simulink model "gxx"  (R2016b)
settings: Solver=VariableStepAuto  StartTime=0.0  StopTime=76  EnableMultiTasking=on
InitFcn:
  | run('motor_param.m')
values from neighbouring files (symbols this model uses):
  battery_Voltage = 390.4254    [motor_param.m]
  Damp = 4.1785e-04    (= 0.00041785)    [motor_param.m]
  Damperr = 0.001    [motor_param.m]
  Inrt = 2.500893701670255e-04    (= 0.000250089370167)    [motor_param.m]
  Pole_pairs = 3    [motor_param.m]
  resistance = 0.11607    [motor_param.m]
  stator_phase_resistance = 0.049039279360294    (= 0.0490392793603)    [motor_param.m]
  temp_amb = 27+273    (= 300)    [motor_param.m]
  Ts = 1e-4    (= 0.0001)    [motor_param.m]
undefined symbols (not defined in the file or in its folder): mot
libraries: fl_lib x17, nesl_utility x8, powerlib x8, simulink x4, electricdrivelib x2, spsDrivesPrivateModels x1
settings Model: Creator=thepu  LastModifiedBy=gd7198
settings OptimizationCC: LifeSpan=inf
settings DebuggingCC: SFUnexpectedBacktrackingDiag=warning  SFNoUnconditionalDefaultTransitionDiag=warning  SFExecutionAtInitializationDiag=none
settings GRTTargetCC: TargetLangStandard=C89/C90 (ANSI)  GeneratePreprocessorConditionals=Disable all
settings ConfigComp: CovMetricSettings=dw  CovHtmlReporting=on  CovSaveCumulativeToWorkspaceVar=on  CovSaveSingleToWorkspaceVar=on  CovExternalEMLEnable=off

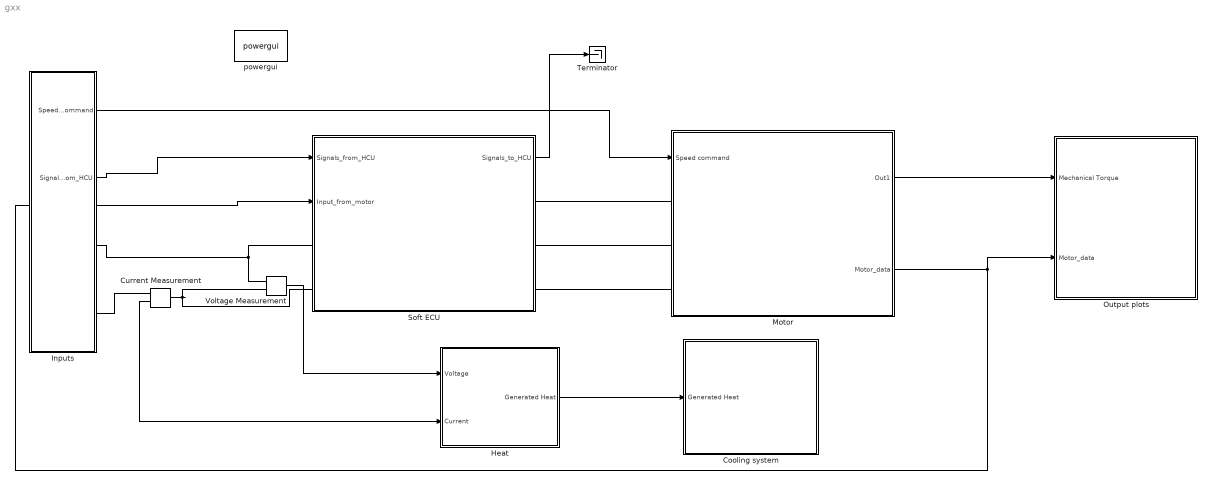
== system gxx ==
  Cooling system : Subsystem
  Current Measurement : powerlib/Measurements/Current Measurement  PhasorSimulation=off  OutputType=Complex  PSBequivalent=0
  Heat : Subsystem
  Inputs : Subsystem
  "Motor " : Subsystem
  Output plots : Subsystem
  Soft ECU : Subsystem
  Terminator : Terminator
  Voltage Measurement : powerlib/Measurements/Voltage Measurement  PhasorSimulation=off  OutputType=Complex  PSBequivalent=0
  powergui : powerlib/powergui  Priority=1  SimulationMode=Discrete  SolverType=Backward Euler  SampleTime=Ts  frequency=60  SPID=off  DisableSnubberDevices=off  DisableRonSwitches=off  DisableVfSwitches=off  SwTol=0  DisplayEquations=off  Interpol=on  ExternalGateDelay=off  methode=off  Ts=10  FunctionMessages=off  echomessages=off  HookPort=off  EnableUseOfTLC=off  x0status=blocks  frequencyindice=0  Pbase=100e6  ErrMax=1e-4  Iterations=50  UnitsV=kV  UnitsW=MW  buscounter=0  RestoreLinks=warning  ResistiveCurrentMeasurement=off  Frange=[0:2:500]  Ylog=off  Xlog=on  ShowGrid=off  save=off  variable=ZData  structure=0  ZoomFFT=off  StartTime=0.0  cycles=1  DisplayStyle=1  fundamental=60  FreqAxis=off  MaxFrequency=1000  frequencyindicesteady=1  RmsSteady=1  display=off
  wires:
  "Motor "/2(Motor_data) -> Soft ECU/2(Input_from_motor), Output plots/2(Motor_data)
  Heat/1(Generated Heat) -> Cooling system/1(Generated Heat)
  Inputs/1(Speed_command) -> "Motor "/1(Speed command)
  "Motor "/1(Out1) -> Output plots/1(Mechanical Torque)
  Inputs/2(Signals_From_HCU) -> Soft ECU/1(Signals_from_HCU)
  Soft ECU/1(Signals_to_HCU) -> Terminator/1
  Voltage Measurement/1 -> Heat/1(Voltage)
  Current Measurement/1 -> Heat/2(Current)
  connections:
  Inputs/RConn1 -- Voltage Measurement/LConn1 -- Soft ECU/LConn1
  "Motor "/LConn1 -- Soft ECU/RConn1
  Soft ECU/RConn2 -- "Motor "/LConn2
  Soft ECU/RConn3 -- "Motor "/LConn3
  Current Measurement/LConn1 -- Voltage Measurement/LConn2 -- Soft ECU/LConn2
  Current Measurement/RConn1 -- Inputs/RConn2

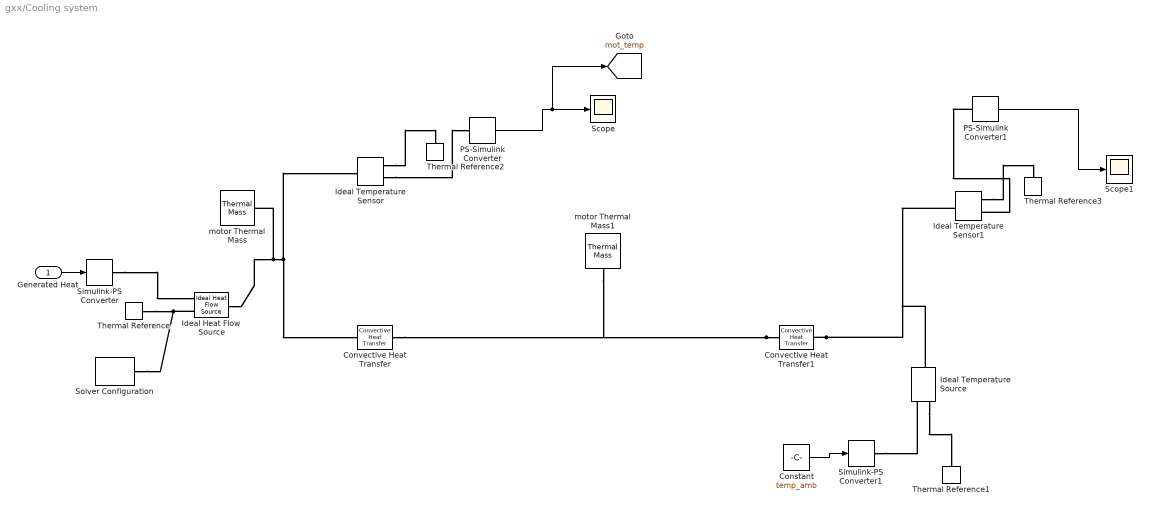
== system gxx/Cooling system ==
  Generated Heat : Inport
  Constant : Constant  Value=temp_amb
  Convective Heat Transfer : fl_lib/Thermal/Thermal Elements/Convective Heat Transfer  area=htArea m^2  heat_tr_coeff=hcm W/(m^2 * K)  Q_specify=off  Q_priority=None  Q=0 J/s  T_specify=off  T_priority=None  T=0 K
  Convective Heat Transfer1 : fl_lib/Thermal/Thermal Elements/Convective Heat Transfer  area=radiator_area m^2  heat_tr_coeff=hac W/(m^2 * K)  Q_specify=off  Q_priority=None  Q=0 J/s  T_specify=off  T_priority=None  T=0 K
  Ideal Heat Flow Source : fl_lib/Thermal/Thermal Sources/Ideal Heat Flow Source
  Ideal Temperature Sensor : fl_lib/Thermal/Thermal Sensors/Ideal Temperature Sensor
  Ideal Temperature Sensor1 : fl_lib/Thermal/Thermal Sensors/Ideal Temperature Sensor
  Ideal Temperature Source : fl_lib/Thermal/Thermal Sources/Ideal Temperature Source
  PS-Simulink Converter : nesl_utility/PS-Simulink Converter  PhysicalDomain=network_engine_domain  SubClassName=ps_output  LeftPortType=input  RightPortType=output  PseudoPeriodic=off  Frequencies=[]  Unit=K  AffineConversion=off
  PS-Simulink Converter1 : nesl_utility/PS-Simulink Converter  PhysicalDomain=network_engine_domain  SubClassName=ps_output  LeftPortType=input  RightPortType=output  PseudoPeriodic=off  Frequencies=[]  Unit=K  AffineConversion=off
  Scope : Scope
  Scope1 : Scope
  Simulink-PS Converter : nesl_utility/Simulink-PS Converter  PhysicalDomain=network_engine_domain  SubClassName=ps_input  LeftPortType=input  RightPortType=output  PseudoPeriodic=off  Frequencies=[]  NoiseDistribution=none  NoiseParameters=[]  Unit=1  AffineConversion=off  InputFiltering=off  SimscapeFilterOrder=1  InputFilterTimeConstant=0.001  UdotUserProvided=1
  Simulink-PS Converter1 : nesl_utility/Simulink-PS Converter  PhysicalDomain=network_engine_domain  SubClassName=ps_input  LeftPortType=input  RightPortType=output  PseudoPeriodic=off  Frequencies=[]  NoiseDistribution=none  NoiseParameters=[]  Unit=K  AffineConversion=off  InputFiltering=off  SimscapeFilterOrder=1  InputFilterTimeConstant=0.001  UdotUserProvided=1
  Solver Configuration : nesl_utility/Solver Configuration  PhysicalDomain=network_engine_domain  SubClassName=solver  LeftPortType=input  RightPortType=generic  Accelerate=off  Tones=[]  Harmonics=[]  SimulateNoise=off  Profile=off  UseLocalSampling=off  EnableSwitchedLinearOptims=on  FrequencyDomain=off  UseCCode=off  RelTol=0.001  AbsTol=1e-06  MinStep=1e-09  ToWorkspace=off  RevertToSquareIcSolve=off  NumHomotopyIterations=100  PhasorMode=off  PhasorModeNumHarmonics=1  OverrideAbsTol=off  DoDC=off  ResidualTolerance=1e-9  UseLocalSolver=off  LocalSolverChoice=NE_BACKWARD_EULER_ADVANCER  LocalSolverSampleTime=0.1  DoFixedCost=off  MaxNonlinIter=3  MaxModeIter=2  LinearAlgebra=Sparse  DelaysMemoryBudget=1024  AutomaticFiltering=on  FilteringTimeConstant=0.001
  Thermal Reference{,1..3} (4 alike) : fl_lib/Thermal/Thermal Elements/Thermal Reference
  motor Thermal Mass : fl_lib/Thermal/Thermal Elements/Thermal Mass  mass=motor_mass kg  sp_heat=motor_cp J/kg/K  T_specify=on  T_priority=High  T=temp_amb K  Q_specify=off  Q_priority=High  Q=0 J/s
  motor Thermal Mass1 : fl_lib/Thermal/Thermal Elements/Thermal Mass  mass=coolant_mass kg  sp_heat=coolant_cp J/kg/K  T_specify=on  T_priority=High  T=temp_amb degC  Q_specify=off  Q_priority=High  Q=0 J/s
  tag scope: mot_temp=global
  wires:
  Generated Heat/1 -> Simulink-PS Converter/1
  Constant/1 -> Simulink-PS Converter1/1
  PS-Simulink Converter/1 -> [mot_temp], Scope/1
  PS-Simulink Converter1/1 -> Scope1/1
  connections:
  Thermal Reference/LConn1 -- Solver Configuration/RConn1 -- Ideal Heat Flow Source/RConn2
  Ideal Heat Flow Source/LConn1 -- motor Thermal Mass/LConn1 -- Ideal Temperature Sensor/LConn1 -- Convective Heat Transfer/LConn1
  Simulink-PS Converter/RConn1 -- Ideal Heat Flow Source/RConn1
  Convective Heat Transfer1/LConn1 -- Convective Heat Transfer/RConn1 -- motor Thermal Mass1/LConn1
  Convective Heat Transfer1/RConn1 -- Ideal Temperature Source/LConn1 -- Ideal Temperature Sensor1/LConn1
  Simulink-PS Converter1/RConn1 -- Ideal Temperature Source/RConn1
  Ideal Temperature Source/RConn2 -- Thermal Reference1/LConn1
  Ideal Temperature Sensor/RConn1 -- Thermal Reference2/LConn1
  Ideal Temperature Sensor/RConn2 -- PS-Simulink Converter/LConn1
  Ideal Temperature Sensor1/RConn1 -- Thermal Reference3/LConn1
  PS-Simulink Converter1/LConn1 -- Ideal Temperature Sensor1/RConn2

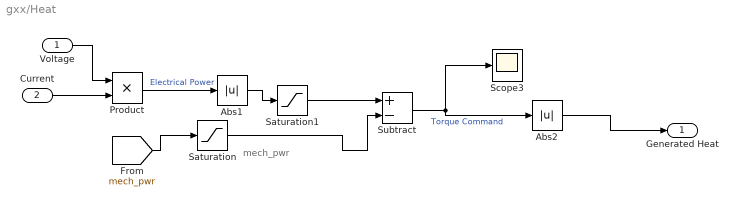
== system gxx/Heat ==
  note: mech_pwr
  Voltage : Inport
  Current : Inport  Port=2
  Abs1 : Abs
  Abs2 : Abs
  Product : Product
  Saturation : Saturate  UpperLimit=100000  LowerLimit=-100000
  Saturation1 : Saturate  UpperLimit=1000000  LowerLimit=-1000000
  Scope3 : Scope
  Subtract : Sum  Inputs=+-
  Generated Heat : Outport
  wires:
  Voltage/1 -> Product/1
  [mech_pwr] -> Saturation/1
  Abs1/1 -> Saturation1/1
  Product/1 -> Abs1/1  "Electrical Power"
  Saturation/1 -> Subtract/2
  Subtract/1 -> Scope3/1, Abs2/1  "Torque Command"
  Abs2/1 -> Generated Heat/1
  Saturation1/1 -> Subtract/1
  Current/1 -> Product/2

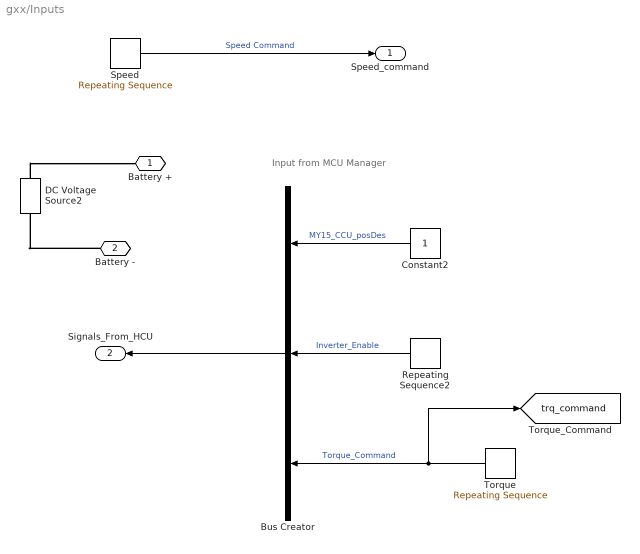
== system gxx/Inputs ==
  note: Input from MCU Manager
  Bus Creator : BusCreator  Inputs=3
  Constant2 : Constant
  DC Voltage Source2 : powerlib/Electrical Sources/DC Voltage Source  Amplitude=battery_Voltage  Measurements=Voltage
  Repeating Sequence2 : simulink/Sources/Repeating Sequence  rep_seq_t=time_test  rep_seq_y=inverterEnable
  Speed : simulink/Sources/Repeating Sequence  rep_seq_t=time_test  rep_seq_y=spd_command
  Torque : simulink/Sources/Repeating Sequence  rep_seq_t=time_test  rep_seq_y=trq_command
  Battery + : PMIOPort  Port=1  Side=Right
  Battery - : PMIOPort  Port=2  Side=Right
  Speed_command : Outport
  Signals_From_HCU : Outport  Port=2
  tag scope: trq_command=global
  wires:
  Speed/1 -> Speed_command/1  "Speed Command"
  Bus Creator/1 -> Signals_From_HCU/1
  Torque/1 -> Bus Creator/3, [trq_command]  "Torque_Command"
  Repeating Sequence2/1 -> Bus Creator/2  "Inverter_Enable"
  Constant2/1 -> Bus Creator/1  "MY15_CCU_posDes"
  connections:
  Battery -/RConn1 -- DC Voltage Source2/LConn1
  DC Voltage Source2/RConn1 -- Battery +/RConn1

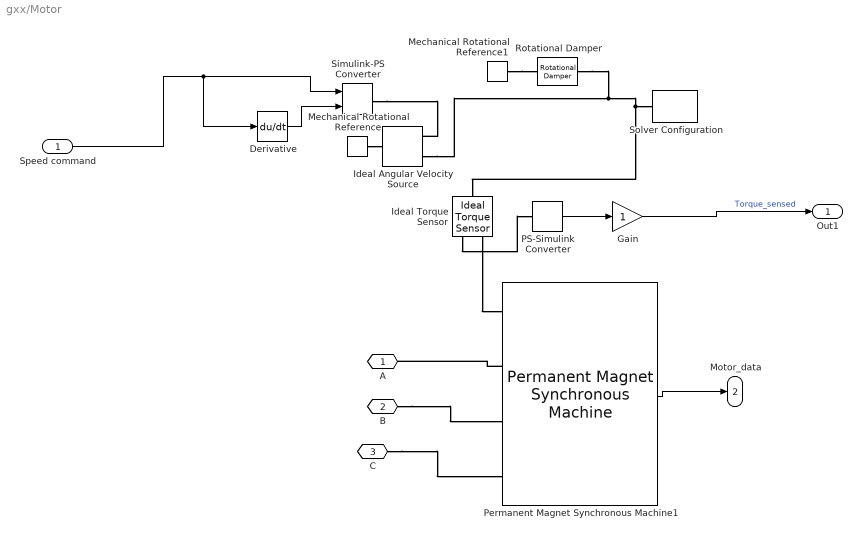
== system gxx/Motor  ==
  Speed command : Inport
  Derivative : Derivative
  Gain : Gain
  Ideal Angular Velocity Source : fl_lib/Mechanical/Mechanical Sources/Ideal Angular Velocity Source
  Ideal Torque Sensor : fl_lib/Mechanical/Mechanical Sensors/Ideal Torque Sensor
  Mechanical Rotational Reference : fl_lib/Mechanical/Rotational Elements/Mechanical Rotational Reference
  Mechanical Rotational Reference1 : fl_lib/Mechanical/Rotational Elements/Mechanical Rotational Reference
  PS-Simulink Converter : nesl_utility/PS-Simulink Converter  PhysicalDomain=network_engine_domain  SubClassName=ps_output  LeftPortType=input  RightPortType=output  PseudoPeriodic=off  Frequencies=[]  Unit=N*m  AffineConversion=off
  Permanent Magnet Synchronous Machine1 : powerlib/Machines/Permanent Magnet Synchronous Machine  NbPhases=3  FluxDistribution=Sinusoidal  RotorType=Round  MechanicalLoad=Mechanical rotational port  PresetModel=No  ShowDetailedParameters=on  MeasurementBus=off  Resistance=stator_phase_resistance  Inductance=8.5e-3  dqInductances=[8.5e-3,8.5e-3]  La=armature_inductance  MachineConstant=Flux linkage established by magnets (V.s)  Flux=flux_linkage  VoltageCst=93.6791  TorqueCst=0.77472  Flat=120  Mechanical=[Inrt Damp Pole_pairs 0]  PolePairs=10  InitialConditions=[0,0, 0,0]  InitialConditions5ph=[0 0 0 0 0 0]  TsPowergui=0  TsBlock=-1  RefAngle=90 degrees behind phase A axis (modified Park)
  Rotational Damper : fl_lib/Mechanical/Rotational Elements/Rotational Damper  D=Damperr N*m/(rad/s)  w_specify=off  w_priority=None  w=0 rad/s  t_specify=off  t_priority=None  t=0 N*m
  Simulink-PS Converter : nesl_utility/Simulink-PS Converter  PhysicalDomain=network_engine_domain  SubClassName=ps_input  LeftPortType=input  RightPortType=output  PseudoPeriodic=off  Frequencies=[]  NoiseDistribution=none  NoiseParameters=[]  Unit=rpm  AffineConversion=off  InputFiltering=derivs  SimscapeFilterOrder=1  InputFilterTimeConstant=0.001  UdotUserProvided=1
  Solver Configuration : nesl_utility/Solver Configuration  PhysicalDomain=network_engine_domain  SubClassName=solver  LeftPortType=input  RightPortType=generic  Accelerate=off  Tones=[]  Harmonics=[]  SimulateNoise=off  Profile=off  UseLocalSampling=off  EnableSwitchedLinearOptims=on  FrequencyDomain=off  UseCCode=off  RelTol=0.001  AbsTol=1e-06  MinStep=1e-09  ToWorkspace=off  RevertToSquareIcSolve=off  NumHomotopyIterations=100  PhasorMode=off  PhasorModeNumHarmonics=1  OverrideAbsTol=off  DoDC=off  ResidualTolerance=1e-09  UseLocalSolver=off  LocalSolverChoice=NE_BACKWARD_EULER_ADVANCER  LocalSolverSampleTime=0.001  DoFixedCost=off  MaxNonlinIter=3  MaxModeIter=2  LinearAlgebra=Sparse  DelaysMemoryBudget=1024  AutomaticFiltering=on  FilteringTimeConstant=0.001
  A : PMIOPort  Port=1  Side=Left
  B : PMIOPort  Port=2  Side=Left
  C : PMIOPort  Port=3  Side=Left
  Out1 : Outport
  Motor_data : Outport  Port=2
  wires:
  Gain/1 -> Out1/1  "Torque_sensed"
  Speed command/1 -> Simulink-PS Converter/1, Derivative/1
  Permanent Magnet Synchronous Machine1/1 -> Motor_data/1
  Derivative/1 -> Simulink-PS Converter/2
  PS-Simulink Converter/1 -> Gain/1
  connections:
  Permanent Magnet Synchronous Machine1/LConn2 -- A/RConn1
  B/RConn1 -- Permanent Magnet Synchronous Machine1/LConn3
  Simulink-PS Converter/RConn1 -- Ideal Angular Velocity Source/RConn1
  Mechanical Rotational Reference1/LConn1 -- Rotational Damper/LConn1
  Ideal Torque Sensor/RConn2 -- PS-Simulink Converter/LConn1
  Mechanical Rotational Reference/LConn1 -- Ideal Angular Velocity Source/LConn1
  Ideal Angular Velocity Source/RConn2 -- Rotational Damper/RConn1 -- Ideal Torque Sensor/LConn1 -- Solver Configuration/RConn1
  C/RConn1 -- Permanent Magnet Synchronous Machine1/LConn4
  Ideal Torque Sensor/RConn1 -- Permanent Magnet Synchronous Machine1/LConn1

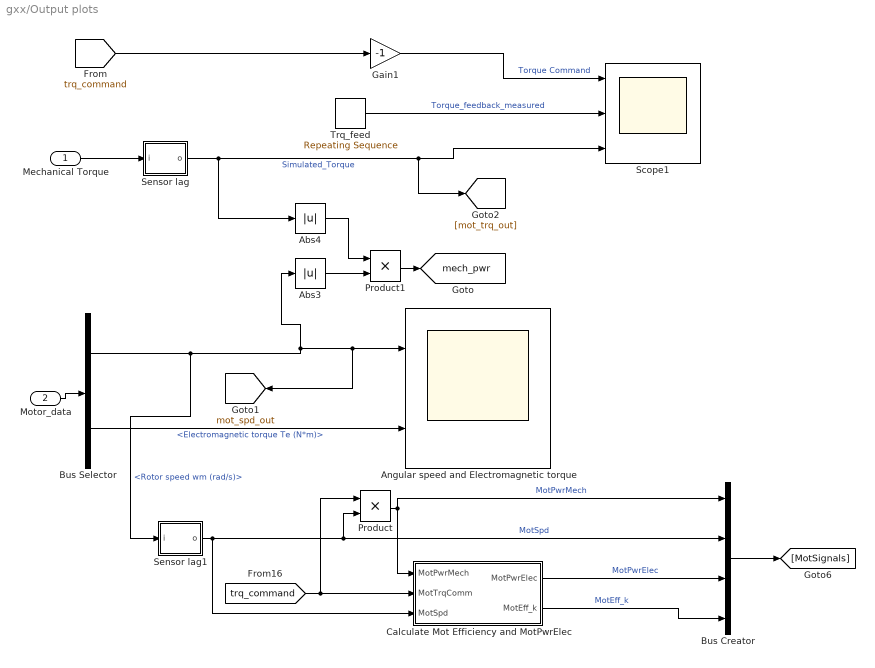
== system gxx/Output plots ==
  Mechanical Torque : Inport
  Motor_data : Inport  Port=2
  Abs3 : Abs
  Abs4 : Abs
  Angular speed and Electromagnetic torque : Scope  NumInputPorts=2
  Bus Creator : BusCreator  Inputs=4
  Bus Selector : BusSelector  OutputSignals=Rotor speed wm (rad/s),Electromagnetic torque Te (N*m)
  Calculate Mot Efficiency and MotPwrElec : Subsystem
  Gain1 : Gain  Gain=-1
  Product : Product
  Product1 : Product
  Scope1 : Scope  NumInputPorts=3
  Sensor lag : Subsystem
  Sensor lag1 : Subsystem
  Trq_feed : simulink/Sources/Repeating Sequence  rep_seq_t=time_test  rep_seq_y=trq_feed
  tag scope: mech_pwr=global, mot_spd_out=global
  wires:
  Bus Selector/1 -> Sensor lag1/1(i), Abs3/1, [mot_spd_out], Angular speed and Electromagnetic torque/1  "<Rotor speed wm (rad/s)>"
  Gain1/1 -> Scope1/1  "Torque Command"
  Abs3/1 -> Product1/2
  Abs4/1 -> Product1/1
  Product1/1 -> [mech_pwr]
  Sensor lag/1(o) -> Abs4/1, [mot_trq_out], Scope1/3  "Simulated_Torque"
  Mechanical Torque/1 -> Sensor lag/1(i)
  Motor_data/1 -> Bus Selector/1
  [trq_command] -> Gain1/1
  Bus Selector/2 -> Angular speed and Electromagnetic torque/2  "<Electromagnetic torque Te (N*m)>"
  Trq_feed/1 -> Scope1/2  "Torque_feedback_measured"
  Bus Creator/1 -> [MotSignals]
  [trq_command] -> Product/1, Calculate Mot Efficiency and MotPwrElec/2(MotTrqComm)
  Sensor lag1/1(o) -> Bus Creator/2, Product/2, Calculate Mot Efficiency and MotPwrElec/3(MotSpd)  "MotSpd"
  Product/1 -> Bus Creator/1, Calculate Mot Efficiency and MotPwrElec/1(MotPwrMech)  "MotPwrMech"
  Calculate Mot Efficiency and MotPwrElec/1(MotPwrElec) -> Bus Creator/3  "MotPwrElec"
  Calculate Mot Efficiency and MotPwrElec/2(MotEff_k) -> Bus Creator/4  "MotEff_k"

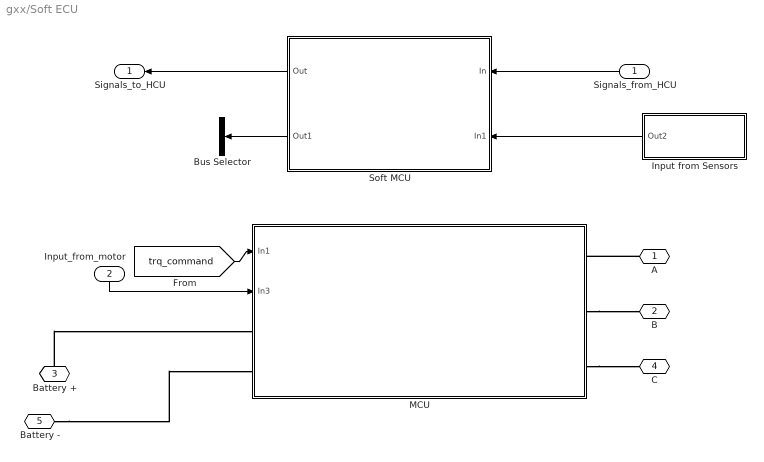
== system gxx/Soft ECU ==
  Signals_from_HCU : Inport
  Input_from_motor : Inport  Port=2
  Bus Selector : BusSelector  OutputSignals=Torque_Command
  Input from Sensors : Subsystem
  MCU : Subsystem
      mask Display: image(imread('MCU.jpg'),'center')
  Soft MCU : Subsystem
      mask Display: image('softECU.jpg')
  A : PMIOPort  Port=1  Side=Right
  B : PMIOPort  Port=2  Side=Right
  Battery + : PMIOPort  Port=3  Side=Left
  C : PMIOPort  Port=4  Side=Right
  Battery - : PMIOPort  Port=5  Side=Left
  Signals_to_HCU : Outport
  wires:
  Signals_from_HCU/1 -> Soft MCU/1(In)
  Soft MCU/1(Out) -> Signals_to_HCU/1
  Input_from_motor/1 -> MCU/2(In3)
  Soft MCU/2(Out1) -> Bus Selector/1
  Input from Sensors/1(Out2) -> Soft MCU/2(In1)
  [trq_command] -> MCU/1(In1)
  connections:
  MCU/RConn2 -- B/RConn1
  MCU/RConn3 -- C/RConn1
  A/RConn1 -- MCU/RConn1
  Battery +/RConn1 -- MCU/LConn1
  Battery -/RConn1 -- MCU/LConn2

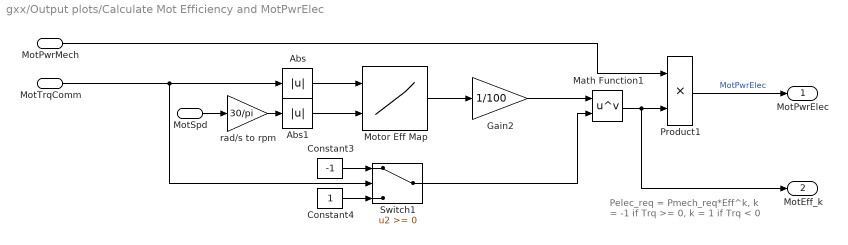
== system gxx/Output plots/Calculate Mot Efficiency and MotPwrElec ==
  note: Pelec_req = Pmech_req*Eff^k,
      | k = -1 if Trq >= 0,
      | k = 1 if Trq < 0
  MotPwrMech : Inport
  MotTrqComm : Inport  Port=2
  MotSpd : Inport  Port=3
  Abs : Abs
  Abs1 : Abs
  Constant3 : Constant  Value=-1  SampleTime=-1
  Constant4 : Constant  SampleTime=-1
  Gain2 : Gain  Gain=1/100
  Math Function1 : Math  Operator=pow  SaturateOnIntegerOverflow=on
  Motor Eff Map : Lookup_n-D  BreakpointsForDimension1=mot.plant.init.eff_trq.idx2_trq  BreakpointsForDimension2=mot.plant.init.eff_trq.idx1_spd  Table=mot.plant.init.eff_trq.map  ExtrapMethod=Clip  UseLastTableValue=on  InternalRulePriority=Speed  RndMeth=Simplest  InputSameDT=on
  Product1 : Product
  Switch1 : Switch
  rad/s to rpm : Gain  Gain=30/pi
  MotPwrElec : Outport
  MotEff_k : Outport  Port=2
  wires:
  Constant3/1 -> Switch1/1
  rad/s to rpm/1 -> Abs1/1
  Abs1/1 -> Motor Eff Map/2
  Constant4/1 -> Switch1/3
  Switch1/1 -> Math Function1/2
  Abs/1 -> Motor Eff Map/1
  Gain2/1 -> Math Function1/1
  Motor Eff Map/1 -> Gain2/1
  Product1/1 -> MotPwrElec/1  "MotPwrElec"
  MotSpd/1 -> rad/s to rpm/1
  Math Function1/1 -> MotEff_k/1, Product1/2
  MotTrqComm/1 -> Abs/1, Switch1/2
  MotPwrMech/1 -> Product1/1

== system gxx/Output plots/Sensor lag ==
  i : Inport
  1st Order LPF of 1ms in Discrete Form : DiscreteTransferFcn  Numerator=[0.6321]  Denominator=[1 -0.3679]  SampleTime=0.001
  o : Outport
  wires:
  i/1 -> 1st Order LPF of 1ms in Discrete Form/1
  1st Order LPF of 1ms in Discrete Form/1 -> o/1

== system gxx/Output plots/Sensor lag1 ==
  i : Inport
  1st Order LPF of 1ms in Discrete Form : DiscreteTransferFcn  Numerator=[0.6321]  Denominator=[1 -0.3679]  SampleTime=0.001
  o : Outport
  wires:
  i/1 -> 1st Order LPF of 1ms in Discrete Form/1
  1st Order LPF of 1ms in Discrete Form/1 -> o/1

== system gxx/Soft ECU/Input from Sensors ==
  Bus Creator : BusCreator  Inputs=7
  Out2 : Outport
  wires:
  Bus Creator/1 -> Out2/1
  [clt_plant_spd_in] -> Bus Creator/7  "clt_plant_spd_in"
  [mcu_temp] -> Bus Creator/6  "mcu_temp"
  [mot_spd_out] -> Bus Creator/1  "mot_spd_out"
  [mot_crr_out] -> Bus Creator/3  "mot_crr_out"
  [mot_volt_in] -> Bus Creator/4  "mot_volt_in"
  [mot_trq_out] -> Bus Creator/2  "mot_trq_out"
  [mot_temp] -> Bus Creator/5  "mot_temp"

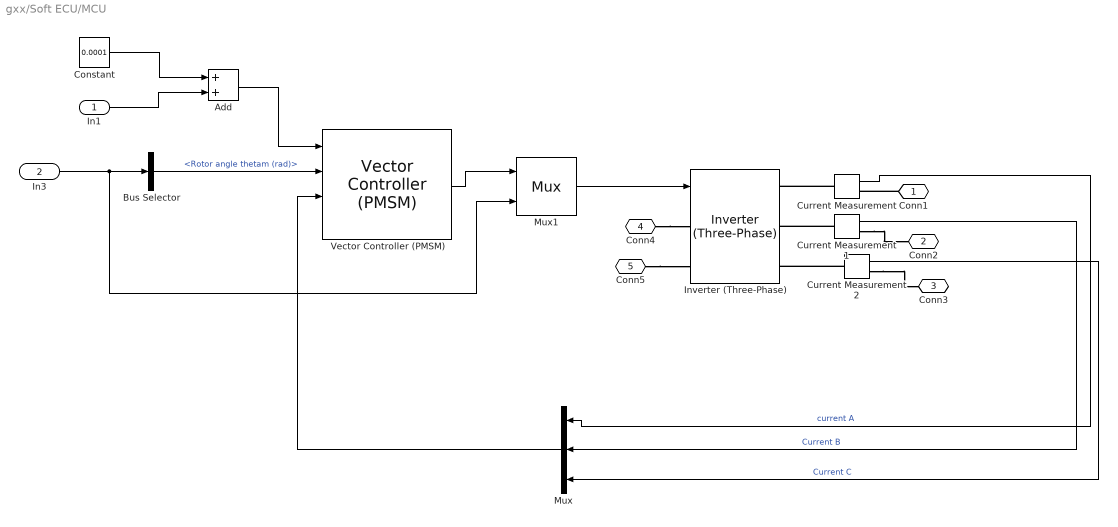
== system gxx/Soft ECU/MCU ==
  In1 : Inport
  In3 : Inport  Port=2
  Add : Sum
  Bus Selector : BusSelector  OutputSignals=Rotor angle thetam (rad)
  Constant : Constant  Value=0.0001
  Current Measurement : powerlib/Measurements/Current Measurement  PhasorSimulation=off  OutputType=Complex  PSBequivalent=0
  Current Measurement1 : powerlib/Measurements/Current Measurement  PhasorSimulation=off  OutputType=Complex  PSBequivalent=0
  Current Measurement2 : powerlib/Measurements/Current Measurement  PhasorSimulation=off  OutputType=Complex  PSBequivalent=0
  Inverter (Three-Phase) : electricdrivelib/Fundamental Drive Blocks/Inverter (Three-Phase)  OverrideUsingVariant=Average_PMSM  detailLevel=Average  driveType=PMSM vector control  Ts=0.1*Ts  SnubberResistance=10e3  SnubberCapacitance=inf  Device=IGBT / Diodes  Ron=Ron  ForwardVoltages=[1.2,1.2]  GTOparameters=[1e-6,2e-6]  IGBTparameters=[1e-6,2e-6]  Measurements=All voltages and currents  converterType=Inverter  SourceFrequency=60  ReferenceFrame=Rotor  dqInductances=[0.0085,0.0085]  Inductance=8.5e-3  Ls=0  Resistance=resistance  Flux=fluxByMagnet  Stator_sm=[2.01e-3,4.289e-4,4.477e-3,1.354e-3]  Stator_im=[14.85e-3,0.3027e-3]  Rotor=[9.295e-3,0.3027e-3]  Lm=10.46e-3  p=Pole_pairs
      link override Average_PMSM/Limit detection/Bus Selector1: OutputSignals=m.Stator current is_d (A),m.Stator current is_q (A),m.Rotor speed wm (rad/s)
      settings: AttributesFormatString=%<BlockChoice>
  Mux : Mux  Inputs=3
  Mux1 : spsDrivesPrivateModels/Mux  OverrideUsingVariant=Average_AC6  detailLevel=Average  driveType=AC6
      settings: AttributesFormatString=%<BlockChoice>
  Vector Controller (PMSM) : electricdrivelib/Fundamental Drive Blocks/Vector Controller (PMSM)  OverrideUsingVariant=Average_3ph  detailLevel=Average  nb_ph=3  modulationType=Hysteresis  Ts_vect=2*Ts  h=0.1  freq_max=20e3  fc_bus=50  car_freq=20000  nb_p=3  machineConstant=Flux linkage established by magnets (V.s)  fluxConstant=0.17197  voltageConstant=126.966  torqueConstant=1.05  kp_Id=200  ki_Id=1000  kp_Iq=200  ki_Iq=1000
      settings: AttributesFormatString=%<BlockChoice>
  Conn1 : PMIOPort  Port=1  Side=Right
  Conn2 : PMIOPort  Port=2  Side=Right
  Conn3 : PMIOPort  Port=3  Side=Right
  Conn4 : PMIOPort  Port=4  Side=Left
  Conn5 : PMIOPort  Port=5  Side=Left
  wires:
  Mux/1 -> Vector Controller (PMSM)/3
  Current Measurement/1 -> Mux/1  "current A"
  Current Measurement1/1 -> Mux/2  "Current B"
  Current Measurement2/1 -> Mux/3  "Current C"
  Mux1/1 -> Inverter (Three-Phase)/1
  In3/1 -> Mux1/2, Bus Selector/1
  Bus Selector/1 -> Vector Controller (PMSM)/2  "<Rotor angle thetam (rad)>"
  Vector Controller (PMSM)/1 -> Mux1/1
  Constant/1 -> Add/1
  In1/1 -> Add/2
  Add/1 -> Vector Controller (PMSM)/1
  connections:
  Conn1/RConn1 -- Current Measurement/RConn1
  Current Measurement2/RConn1 -- Conn3/RConn1
  Current Measurement1/RConn1 -- Conn2/RConn1
  Current Measurement1/LConn1 -- Inverter (Three-Phase)/RConn2
  Current Measurement/LConn1 -- Inverter (Three-Phase)/RConn1
  Current Measurement2/LConn1 -- Inverter (Three-Phase)/RConn3
  Conn4/RConn1 -- Inverter (Three-Phase)/LConn1
  Conn5/RConn1 -- Inverter (Three-Phase)/LConn2

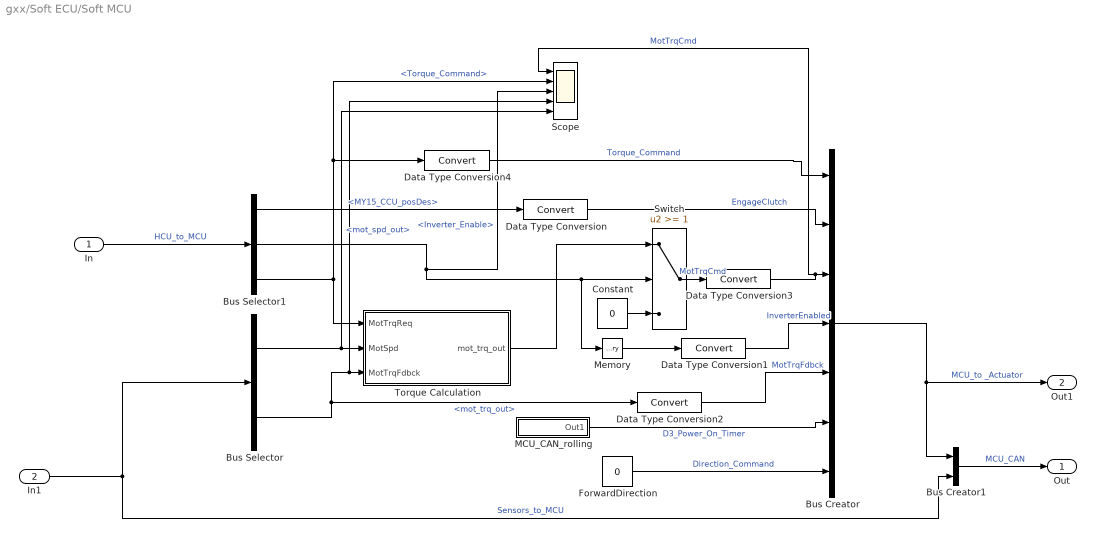
== system gxx/Soft ECU/Soft MCU ==
  In : Inport
  In1 : Inport  Port=2
  Bus Creator : BusCreator  Inputs=7
  Bus Creator1 : BusCreator  Inputs=2
  Bus Selector : BusSelector  OutputSignals=mot_spd_out,mot_trq_out
  Bus Selector1 : BusSelector  OutputSignals=MY15_CCU_posDes,Inverter_Enable,Torque_Command
  Constant : Constant  Value=0
  Data Type Conversion{,1..4} (5 alike) : DataTypeConversion
  ForwardDirection : Constant  Value=0
  MCU_CAN_rolling : Subsystem
  Memory : Memory
  Scope : Scope  NumInputPorts=5
  Switch : Switch  Threshold=1
  Torque Calculation : Subsystem
  Out : Outport
  Out1 : Outport  Port=2
  wires:
  In1/1 -> Bus Creator1/2, Bus Selector/1  "Sensors_to_MCU"
  Bus Creator1/1 -> Out/1  "MCU_CAN"
  In/1 -> Bus Selector1/1  "HCU_to_MCU"
  Bus Selector1/3 -> Data Type Conversion4/1, Scope/2, Torque Calculation/1(MotTrqReq)  "<Torque_Command>"
  Bus Creator/1 -> Bus Creator1/1, Out1/1  "MCU_to _Actuator"
  Bus Selector1/2 -> Memory/1, Switch/2, Scope/3  "<Inverter_Enable>"
  Constant/1 -> Switch/3
  Bus Selector1/1 -> Data Type Conversion/1  "<MY15_CCU_posDes>"
  Data Type Conversion/1 -> Bus Creator/2  "EngageClutch"
  Bus Selector/1 -> Scope/5, Torque Calculation/2(MotSpd)  "<mot_spd_out>"
  Torque Calculation/1(mot_trq_out) -> Switch/1
  Data Type Conversion1/1 -> Bus Creator/4  "InverterEnabled"
  Bus Selector/2 -> Scope/4, Torque Calculation/3(MotTrqFdbck), Data Type Conversion2/1  "<mot_trq_out>"
  Data Type Conversion2/1 -> Bus Creator/5  "MotTrqFdbck"
  Memory/1 -> Data Type Conversion1/1
  Switch/1 -> Data Type Conversion3/1  "MotTrqCmd"
  Data Type Conversion3/1 -> Scope/1, Bus Creator/3  "MotTrqCmd"
  Data Type Conversion4/1 -> Bus Creator/1  "Torque_Command"
  MCU_CAN_rolling/1(Out1) -> Bus Creator/6  "D3_Power_On_Timer"
  ForwardDirection/1 -> Bus Creator/7  "Direction_Command"

== system gxx/Soft ECU/Soft MCU/MCU_CAN_rolling ==
  Constant8 : Constant
  Rolling Alive Counter1 : Stateflow chart  TreatAsAtomicUnit=on
  Switch1 : Switch  Criteria=u2 > Threshold
  Out1 : Outport
  wires:
  Switch1/1 -> Out1/1  "MCURollingAliveCnt [0 1 2 3]"
  [MCU_CAN_fault] -> Switch1/2
  Constant8/1 -> Switch1/1
  Rolling Alive Counter1/1(RollingAliveCnt) -> Switch1/3

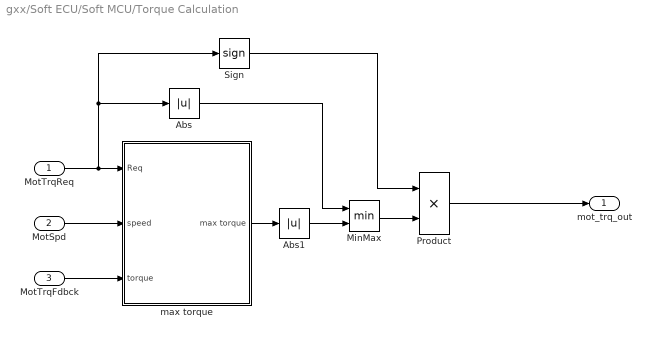
== system gxx/Soft ECU/Soft MCU/Torque Calculation ==
  MotTrqReq : Inport
  MotSpd : Inport  Port=2
  MotTrqFdbck : Inport  Port=3
  Abs : Abs
  Abs1 : Abs
  MinMax : MinMax  Inputs=2
  Product : Product
  Sign : Signum
  "max torque " : Subsystem
  mot_trq_out : Outport
  wires:
  Product/1 -> mot_trq_out/1
  "max torque "/1(max torque) -> Abs1/1
  MotSpd/1 -> "max torque "/2(speed)
  MotTrqReq/1 -> "max torque "/1(Req), Sign/1, Abs/1
  Sign/1 -> Product/1
  MinMax/1 -> Product/2
  Abs/1 -> MinMax/1
  Abs1/1 -> MinMax/2
  MotTrqFdbck/1 -> "max torque "/3(torque)

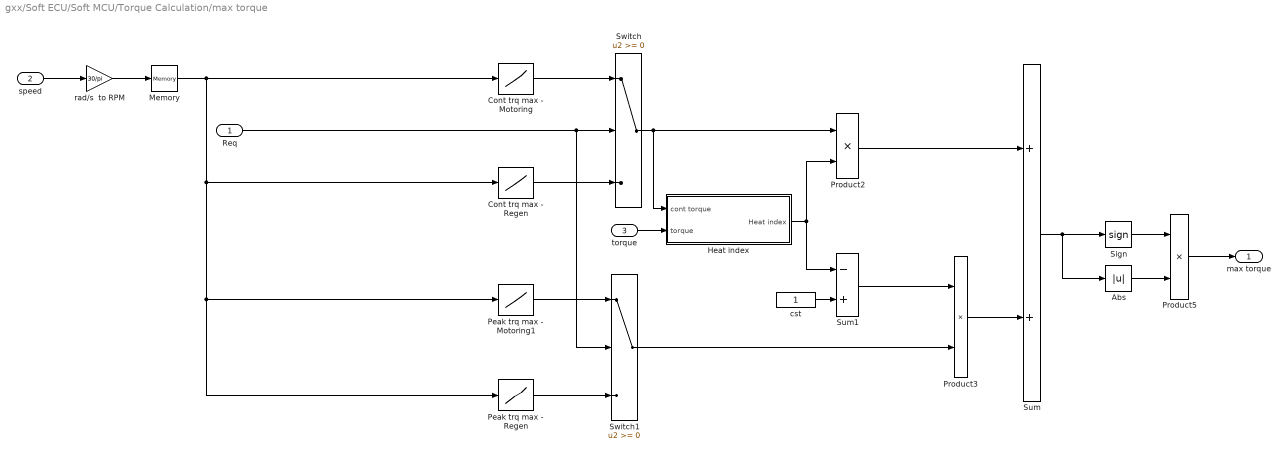
== system gxx/Soft ECU/Soft MCU/Torque Calculation/max torque  ==
  Req : Inport
  speed : Inport  Port=2
  torque : Inport  Port=3
  Abs : Abs  SaturateOnIntegerOverflow=on
  Cont trq max - Motoring : Lookup  InputValues=mot.plant.init.motor.trq_cont.idx1_spd  Table=mot.plant.init.motor.trq_cont.map  LookUpMeth=Interpolation-Use End Values  SaturateOnIntegerOverflow=on
  Cont trq max - Regen : Lookup  InputValues=mot.plant.init.regen.trq_cont.idx1_spd  Table=mot.plant.init.regen.trq_cont.map  LookUpMeth=Interpolation-Use End Values  SaturateOnIntegerOverflow=on
  Heat index : Subsystem
  Memory : Memory
  Peak trq max - Motoring1 : Lookup  InputValues=mot.plant.init.regen.trq_max.idx1_spd  Table=mot.plant.init.motor.trq_max.map  LookUpMeth=Interpolation-Use End Values  SaturateOnIntegerOverflow=on
  Peak trq max - Regen : Lookup  InputValues=mot.plant.init.regen.trq_max.idx1_spd  Table=mot.plant.init.regen.trq_max.map  LookUpMeth=Interpolation-Use End Values  SaturateOnIntegerOverflow=on
  Product2 : Product  SaturateOnIntegerOverflow=on  InputSameDT=on  OutDataTypeStr=Inherit: Same as first input
  Product3 : Product  SaturateOnIntegerOverflow=on  InputSameDT=on  OutDataTypeStr=Inherit: Same as first input
  Product5 : Product  SaturateOnIntegerOverflow=on  InputSameDT=on  OutDataTypeStr=Inherit: Same as first input
  Sign : Signum
  Sum : Sum  SaturateOnIntegerOverflow=on  InputSameDT=on  OutDataTypeStr=Inherit: Same as first input
  Sum1 : Sum  Inputs=-+  SaturateOnIntegerOverflow=on  InputSameDT=on  OutDataTypeStr=Inherit: Same as first input
  Switch : Switch  SaturateOnIntegerOverflow=on
  Switch1 : Switch  SaturateOnIntegerOverflow=on
  cst : Constant
  rad/s  to RPM : Gain  Gain=30/pi
  max torque : Outport
  wires:
  Heat index/1(Heat index) -> Product2/2, Sum1/1
  cst/1 -> Sum1/2
  Product3/1 -> Sum/2
  Sum1/1 -> Product3/1
  Product2/1 -> Sum/1
  Switch1/1 -> Product3/2
  Switch/1 -> Heat index/1(cont torque), Product2/1
  Peak trq max - Regen/1 -> Switch1/3
  Cont trq max - Regen/1 -> Switch/3
  Cont trq max - Motoring/1 -> Switch/1
  speed/1 -> rad/s  to RPM/1
  torque/1 -> Heat index/2(torque)
  Abs/1 -> Product5/2
  Sum/1 -> Abs/1, Sign/1
  Product5/1 -> max torque/1
  Sign/1 -> Product5/1
  Memory/1 -> Cont trq max - Motoring/1, Cont trq max - Regen/1, Peak trq max - Motoring1/1, Peak trq max - Regen/1
  rad/s  to RPM/1 -> Memory/1
  Req/1 -> Switch/2, Switch1/2
  Peak trq max - Motoring1/1 -> Switch1/1

== system gxx/Soft ECU/Soft MCU/Torque Calculation/max torque /Heat index ==
  note: Heat index calculation
  cont torque : Inport
  torque : Inport  Port=2
  Abs : Abs  SaturateOnIntegerOverflow=on
  Divide : Subsystem  mask(Divide){}
      mask Display: disp('Divide')
  Heat Energy Factor : Integrator  InitialCondition=-0.3  LimitOutput=on  UpperSaturationLimit=1  LowerSaturationLimit=-0.3
  Heating Constant : Gain  Gain=0.3/mot.plant.init.t_max_trq  SaturateOnIntegerOverflow=on  OutDataTypeStr=Inherit: Same as input  ParamDataTypeStr=Inherit: Same as input
  Saturation : Saturate  UpperLimit=1  LowerLimit=0
  Sum : Sum  Inputs=+-  SaturateOnIntegerOverflow=on  InputSameDT=on  OutDataTypeStr=Inherit: Same as first input
  motor inertia (Nms^2\rad)5 : Constant
  Heat index : Outport
  wires:
  cont torque/1 -> Divide/2(denominator)
  Abs/1 -> Sum/1
  Saturation/1 -> Heat index/1
  motor inertia (Nms^2\rad)5/1 -> Sum/2
  Divide/1(quotient) -> Abs/1
  Sum/1 -> Heating Constant/1
  Heating Constant/1 -> Heat Energy Factor/1
  Heat Energy Factor/1 -> Saturation/1
  torque/1 -> Divide/1(numerator)

== system gxx/Soft ECU/Soft MCU/Torque Calculation/max torque /Heat index/Divide ==
  note: Take care of
      | division by 0
  numerator : Inport
  denominator : Inport  Port=2
  Fcn : Fcn  Expr=u[1] / ( u[2] + eps*(u[2]==0) )
  Mux : Mux  Inputs=2
  quotient : Outport
  wires:
  denominator/1 -> Mux/2
  Fcn/1 -> quotient/1
  numerator/1 -> Mux/1
  Mux/1 -> Fcn/1

== stateflow chart gxx/Soft ECU/Soft MCU/MCU_CAN_rolling/Rolling Alive Counter1 ==
  state RollingAliveCounter
    state Count1
      en: RollingAliveCnt=0;
    state Count2
      en: RollingAliveCnt=1;
    state Count3
      en: RollingAliveCnt=2;
    state Count4
      en: RollingAliveCnt=3;
    (default) -> Count1
    Count4 -> Count1 : after(0.01,sec)
    Count1 -> Count2 : after(0.01,sec)
    Count2 -> Count3 : after(0.01,sec)
    Count3 -> Count4 : after(0.01,sec)
  data: RollingAliveCnt output double
